simulink model "simulation3Phase"  (R2014a)
settings: Solver=ode23s  StartTime=0.0  StopTime=5  FixedStep=0.001  MaxStep=0.0001  RelTol=1e-2
libraries: powerlib x26, powerlib_meascontrol x8, simulink x1
settings Model: Creator=User  LastModifiedBy=Bauyrzhan
settings DebuggingCC: UnderspecifiedInitializationDetection=Classic

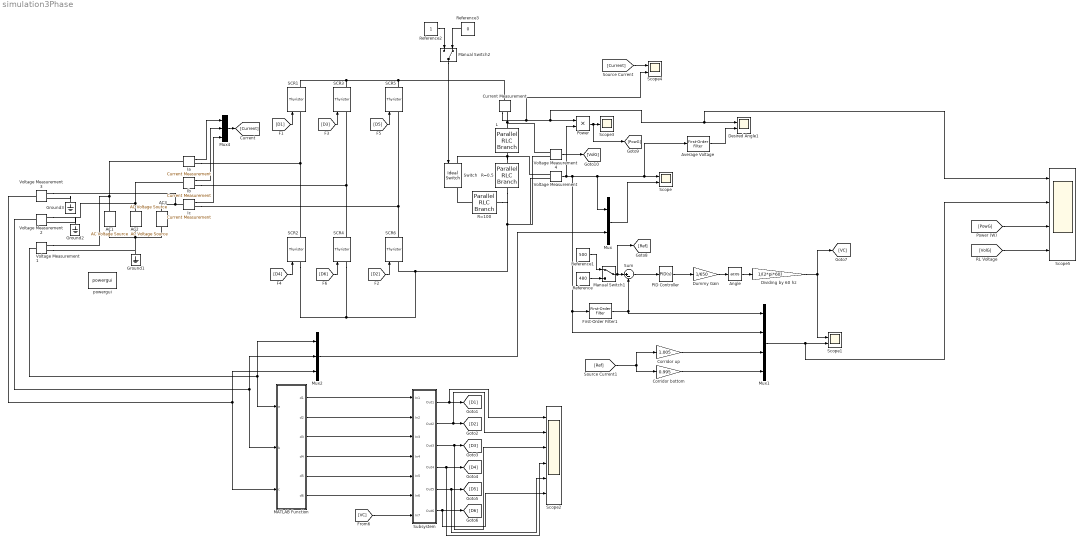
== system simulation3Phase ==
  AC1 : powerlib/Electrical Sources/AC Voltage Source  Amplitude=678.82  Phase=0  Frequency=60  SampleTime=0  Measurements=None
  AC2 : powerlib/Electrical Sources/AC Voltage Source  Amplitude=678.82  Phase=240  Frequency=60  SampleTime=0  Measurements=None
  AC3 : powerlib/Electrical Sources/AC Voltage Source  Amplitude=678.82  Phase=120  Frequency=60  SampleTime=0  Measurements=None
  Angle : Trigonometry  Operator=acos
  Average Voltage : powerlib_meascontrol/Filters/First-Order Filter  FilterType=Lowpass  Tc=1/60  Ts=0  Initialize=on  Vac_Init=[0, 0, 60]  Vdc_Init=0  PlotResponse=off  FreqRange="[0,  200,  1]"
  Corridor bottom : Gain  Gain=0.995
  Corridor up : Gain  Gain=1.005
  Current Measurement : powerlib/Measurements/Current Measurement  PhasorSimulation=off  OutputType=Complex  PSBequivalent=0
  Desired Angle1 : Scope  NumInputPorts=2
      settings: ShowLegends=on  YMin=-50~-25  YMax=1050~525  SaveName=ScopeData5
  Dividing by 60 hz : Gain  Gain=1/(2*pi*60)
  Dummy Gain : Gain  Gain=1/650
  First-Order Filter1 : powerlib_meascontrol/Filters/First-Order Filter  FilterType=Lowpass  Tc=2e-5  Ts=0  Initialize=on  Vac_Init=[0, 0, 60]  Vdc_Init=0  PlotResponse=off  FreqRange="[0,  200,  1]"
  Ground1 : powerlib/Elements/Ground  LConnTagsString=a
  Ground2 : powerlib/Elements/Ground  LConnTagsString=a
  Ground3 : powerlib/Elements/Ground  LConnTagsString=a
  Ia : powerlib/Measurements/Current Measurement  PhasorSimulation=off  OutputType=Complex  PSBequivalent=0
  Ib : powerlib/Measurements/Current Measurement  PhasorSimulation=off  OutputType=Complex  PSBequivalent=0
  Ic : powerlib/Measurements/Current Measurement  PhasorSimulation=off  OutputType=Complex  PSBequivalent=0
  L : powerlib/Elements/Parallel RLC Branch  LConnTagsString=a  RConnTagsString=__new0  BranchType=L  Resistance=1  Inductance=0.042  SetiL0=off  InitialCurrent=10000  Capacitance=3000e-6  Setx0=off  InitialVoltage=0  Measurements=None
  MATLAB Function : MATLAB Function  TreatAsAtomicUnit=on
  Manual Switch1 : ManualSwitch
  Manual Switch2 : ManualSwitch  CurrentSetting=0
  Mux : Mux  Inputs=2
  Mux1 : Mux
  Mux2 : Mux  Inputs=3
  Mux4 : Mux  Inputs=3
  PID Controller : simulink/Continuous/PID Controller  Controller=PID  TimeDomain=Continuous-time  SampleTime=1  IntegratorMethod=Forward Euler  FilterMethod=Forward Euler  Form=Parallel  P=50  I=20  D=0  N=100  InitialConditionSource=internal  InitialConditionForIntegrator=0  InitialConditionForFilter=0  ExternalReset=none  LimitOutput=off  UpperSaturationLimit=inf  LowerSaturationLimit=-inf  LinearizeAsGain=on  AntiWindupMode=none  Kb=1  TrackingMode=off  Kt=1  PParamMin=[]  PParamMax=[]  IParamMin=[]  IParamMax=[]  DParamMin=[]  DParamMax=[]  NParamMin=[]  NParamMax=[]  KbParamMin=[]  KbParamMax=[]  KtParamMin=[]  KtParamMax=[]  POutMin=[]  POutMax=[]  IOutMin=[]  IOutMax=[]  DOutMin=[]  DOutMax=[]  NOutMin=[]  NOutMax=[]  KbOutMin=[]  KbOutMax=[]  KtOutMin=[]  KtOutMax=[]  IntegratorOutMin=[]  IntegratorOutMax=[]  FilterOutMin=[]  FilterOutMax=[]  SumOutMin=[]  SumOutMax=[]  SumI1OutMin=[]  SumI1OutMax=[]  SumI2OutMin=[]  SumI2OutMax=[]  SumI3OutMin=[]  SumI3OutMax=[]  SumDOutMin=[]  SumDOutMax=[]  SaturationOutMin=[]  SaturationOutMax=[]  IntegratorContinuousStateAttributes=''  IntegratorStateMustResolveToSignalObject=off  IntegratorRTWStateStorageClass=Auto  FilterContinuousStateAttributes=''  FilterStateMustResolveToSignalObject=off  FilterRTWStateStorageClass=Auto
  Power : Product
  R=0.5 : powerlib/Elements/Parallel RLC Branch  LConnTagsString=a  RConnTagsString=__new0  BranchType=R  Resistance=0.5  Inductance=1e-3  SetiL0=off  InitialCurrent=0  Capacitance=3000e-6  Setx0=off  InitialVoltage=0  Measurements=None
  R=100 : powerlib/Elements/Parallel RLC Branch  LConnTagsString=a  RConnTagsString=__new0  BranchType=R  Resistance=100  Inductance=1e-3  SetiL0=off  InitialCurrent=0  Capacitance=3000e-6  Setx0=off  InitialVoltage=0  Measurements=None
  Reference : Constant  Value=480
  Reference1 : Constant  Value=500
  Reference2 : Constant
  Reference3 : Constant  Value=0
  SCR{1..6} (6 alike) : powerlib/Power Electronics/Thyristor  Ron=0.000001  Lon=0  Vf=0  IC=0  Rs=5000000  Cs=2e-6  Measurements=on
  Scope : Scope  NumInputPorts=2
      settings: YMin=-50~-700  YMax=650~700
  Scope1 : Scope  NumInputPorts=2
      settings: ShowLegends=on  YMin=0.002825~-25  YMax=0.0034~525
  Scope2 : Scope  NumInputPorts=6
      settings: YMin=0.002825~499.3~-5~-5~-5~-5  YMax=0.0034~500.45~5~5~5~5  SaveName=ScopeData6
  Scope3 : Scope
      settings: ShowLegends=on  TimeRange=0.05602233711133542  YMin=498600  YMax=500900  SaveName=ScopeData3
  Scope4 : Scope  NumInputPorts=2
      settings: ShowLegends=on  YMin=-1100~-100  YMax=1100~1200  SaveName=ScopeData4
  Scope5 : Scope  NumInputPorts=4
      settings: ShowLegends=on  YMin=200~-50~0~-200  YMax=1050~650~550000~1200  SaveName=ScopeData8
  Subsystem : Subsystem
  Sum : Sum  Inputs=|+-
  Switch : powerlib/Power Electronics/Ideal Switch  Ron=0.000001  Lon=0  IC=0  Rs=1e5  Cs=inf  Measurements=on
  Voltage Measurement{,1..4} (5 alike) : powerlib/Measurements/Voltage Measurement  PhasorSimulation=off  OutputType=Complex  PSBequivalent=0
  powergui : powerlib/powergui  Priority=1  SimulationMode=Continuous  SolverType=Tustin  SampleTime=50e-6  frequency=60  SPID=off  DisableSnubberDevices=off  DisableRonSwitches=off  DisableVfSwitches=off  SwTol=0  Interpol=off  DisplayEquations=off  Ts=0  methode=off  frequencyindice=0  Pbase=100e6  ErrMax=1e-4  Iterations=50  UnitsV=kV  UnitsW=MW  FunctionMessages=off  echomessages=off  HookPort=off  EnableUseOfTLC=off  x0status=blocks  RestoreLinks=warning  ResistiveCurrentMeasurement=off  Frange=[0:2:500]  Ylog=off  Xlog=on  ShowGrid=off  save=off  variable=ZData  structure=0  ZoomFFT=off  StartTime=0.0  cycles=1  DisplayStyle=1  fundamental=60  FreqAxis=off  MaxFrequency=1000  frequencyindicesteady=1  RmsSteady=1  display=off
  wires:
  Mux/1 -> Scope/2
  [D1] -> SCR1/1
  [D3] -> SCR3/1
  [D5] -> SCR5/1
  [D4] -> SCR2/1
  [D6] -> SCR4/1
  [D2] -> SCR6/1
  Voltage Measurement1/1 -> Mux2/1, MATLAB Function/1(a)
  Voltage Measurement2/1 -> Mux2/2, MATLAB Function/2(b)
  Voltage Measurement3/1 -> Mux2/3, MATLAB Function/3(c)
  [VC] -> Subsystem/7(In7)
  Subsystem/1(Out1) -> Scope2/1, [D1]
  Subsystem/2(Out2) -> Scope2/2, [D2]
  Subsystem/3(Out3) -> Scope2/3, [D3]
  Subsystem/4(Out4) -> Scope2/4, [D4]
  Subsystem/5(Out5) -> Scope2/5, [D5]
  Subsystem/6(Out6) -> Scope2/6, [D6]
  MATLAB Function/1(d1) -> Subsystem/1(In1)
  MATLAB Function/2(d2) -> Subsystem/2(In2)
  MATLAB Function/5(d5) -> Subsystem/5(In5)
  MATLAB Function/6(d6) -> Subsystem/6(In6)
  MATLAB Function/3(d3) -> Subsystem/3(In3)
  MATLAB Function/4(d4) -> Subsystem/4(In4)
  Mux2/1 -> Mux/2
  Voltage Measurement/1 -> Power/2, First-Order Filter1/1, Mux1/2, Mux/1, Average Voltage/1, Scope/1
  Sum/1 -> PID Controller/1
  PID Controller/1 -> Dummy Gain/1
  Dummy Gain/1 -> Angle/1
  Dividing by 60 hz/1 -> [VC], Scope1/1
  Manual Switch1/1 -> [Ref], Sum/1
  Reference/1 -> Manual Switch1/2
  Reference1/1 -> Manual Switch1/1
  First-Order Filter1/1 -> Mux1/1, Sum/2
  Power/1 -> [PowG], Scope3/1
  Ic/1 -> Mux4/3
  Ib/1 -> Mux4/2
  Ia/1 -> Mux4/1
  Mux4/1 -> [Current]
  [Current] -> Scope4/1
  Current Measurement/1 -> Scope4/2, Scope5/1, Desired Angle1/1, Power/1
  Average Voltage/1 -> Desired Angle1/2
  Corridor up/1 -> Mux1/3
  Corridor bottom/1 -> Mux1/4
  [Ref] -> Corridor bottom/1, Corridor up/1
  Voltage Measurement4/1 -> [VolG]
  Mux1/1 -> Scope5/2, Scope1/2
  [PowG] -> Scope5/3
  [VolG] -> Scope5/4
  Angle/1 -> Dividing by 60 hz/1
  Reference3/1 -> Manual Switch2/2
  Reference2/1 -> Manual Switch2/1
  Manual Switch2/1 -> Switch/1
  connections:
  Voltage Measurement3/LConn1 -- AC3/RConn1 -- Ic/LConn1
  SCR4/RConn1 -- SCR3/LConn1 -- Ib/RConn1
  AC2/LConn1 -- Voltage Measurement1/LConn2 -- Ground1/LConn1 -- AC1/LConn1 -- AC3/LConn1
  SCR2/LConn1 -- SCR4/LConn1 -- Voltage Measurement/LConn2 -- Voltage Measurement4/LConn2 -- R=0.5/RConn1 -- R=100/RConn1 -- SCR6/LConn1
  SCR1/RConn1 -- SCR3/RConn1 -- Current Measurement/LConn1 -- SCR5/RConn1
  Ground3/LConn1 -- Voltage Measurement3/LConn2
  Ground2/LConn1 -- Voltage Measurement2/LConn2
  Voltage Measurement4/LConn1 -- L/LConn1 -- Current Measurement/RConn1
  SCR2/RConn1 -- SCR1/LConn1 -- Ia/RConn1
  SCR6/RConn1 -- SCR5/LConn1 -- Ic/RConn1
  Voltage Measurement2/LConn1 -- Ib/LConn1 -- AC2/RConn1
  Voltage Measurement1/LConn1 -- Ia/LConn1 -- AC1/RConn1
  Voltage Measurement/LConn1 -- Switch/LConn1 -- L/RConn1 -- R=0.5/LConn1
  R=100/LConn1 -- Switch/RConn1

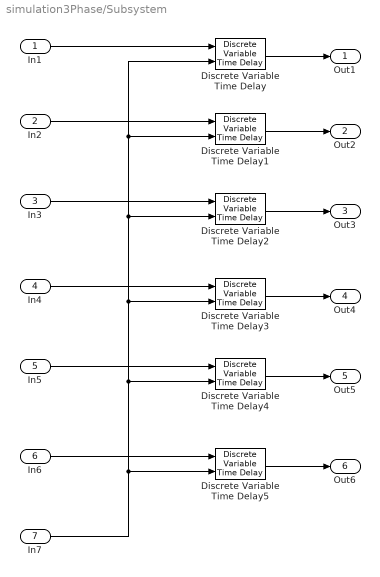
== system simulation3Phase/Subsystem ==
  In1 : Inport
  In2 : Inport  Port=2
  In3 : Inport  Port=3
  In4 : Inport  Port=4
  In5 : Inport  Port=5
  In6 : Inport  Port=6
  In7 : Inport  Port=7
  Discrete Variable Time Delay{,1..5} (6 alike) : powerlib_meascontrol/Additional Components/Discrete Variable Time Delay  MaxDelay=1  InitialValue=0  Ts=50e-6  DFT=on
  Out1 : Outport
  Out2 : Outport  Port=2
  Out3 : Outport  Port=3
  Out4 : Outport  Port=4
  Out5 : Outport  Port=5
  Out6 : Outport  Port=6
  wires:
  In1/1 -> Discrete Variable Time Delay/1
  In2/1 -> Discrete Variable Time Delay1/1
  In7/1 -> Discrete Variable Time Delay5/2, Discrete Variable Time Delay4/2, Discrete Variable Time Delay3/2, Discrete Variable Time Delay2/2, Discrete Variable Time Delay1/2, Discrete Variable Time Delay/2
  In6/1 -> Discrete Variable Time Delay5/1
  In5/1 -> Discrete Variable Time Delay4/1
  In4/1 -> Discrete Variable Time Delay3/1
  In3/1 -> Discrete Variable Time Delay2/1
  Discrete Variable Time Delay/1 -> Out1/1
  Discrete Variable Time Delay1/1 -> Out2/1
  Discrete Variable Time Delay2/1 -> Out3/1
  Discrete Variable Time Delay3/1 -> Out4/1
  Discrete Variable Time Delay4/1 -> Out5/1
  Discrete Variable Time Delay5/1 -> Out6/1

== matlab function simulation3Phase/MATLAB Function ==
  data: a input; d1 output; b input; c input; d2 output; d3 output; d4 output; d5 output; d6 output
function [d1,d2,d3,d4,d5,d6]= fcn(a,b,c)
%#codegen

d1 = 0;
d2 = 0;
d3 = 0;
d4 = 0;
d5 = 0;
d6 = 0;

ab = 0;
ac = 0;
bc = 0;
ba = 0;
ca = 0;
cb = 0;

Vab = abs(a)+abs(b);
Vac = abs(a)+abs(c);
Vbc = abs(b)+abs(c);

if (Vab>Vac && Vab>Vbc && a>b && a>c)
   ab = 1;
end

if (Vac>Vab && Vac>Vbc && a>b && a>c)
    ac = 1;
end

if (Vbc>Vac && Vbc>Vab && b>a && b>c)
    bc = 1;
end

if (Vab>Vac && Vab>Vbc && b>a && b>c)
   ba = 1;
end

if (Vac>Vab && Vac>Vbc && c>a && c>b)
   ca = 1;
end

if (Vbc>Vac && Vbc>Vab && c>a && c>b)
   cb = 1;
end



if (ab == 1)
    d6 = 1;
    d1 = 1;
end

if (ac == 1)
    d1 = 1;
    d2 = 1;
end

if (bc == 1)
    d2 = 1;
    d3 = 1;
end

if (ba == 1)
   d3 = 1;
   d4 = 1;
end

if (ca == 1)
    d4 = 1;
    d5 = 1;
end

if (cb == 1)
    d5 = 1;
    d6 = 1;
end








end
